simulink model "blockdemo"  (Simulink 6.3)
settings: Solver=ode45  StartTime=0.0  StopTime=30  RelTol=1e-3
InitFcn:
  | %% DSPBuilder Start
  | alt_dspbuilder_update_model(bdroot)
  | %% DSPBuilder End
libraries: allblocks_alteradspbuilder2 x7
settings Model: Creator=cpurcell  LastModifiedBy=delphick
settings DebuggingCC: MultiTaskDSMMsg=error

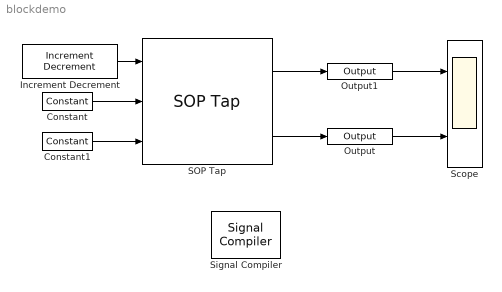
== system blockdemo ==
  Constant : allblocks_alteradspbuilder2/Constant  mask_cst=3.25  BusType=Signed Fractional  bwl=4  bwr=4  SpecifyClock=off
  Constant1 : allblocks_alteradspbuilder2/Constant  mask_cst=-1.75  BusType=Signed Fractional  bwl=4  bwr=4  SpecifyClock=off
  Increment Decrement : allblocks_alteradspbuilder2/Increment Decrement  BusType=Signed Fractional  bwl=2  bwr=2  SpecifyClock=off  clr_value=0  direction=Increment  phase_selection=1  use_ena=off  use_sclr=off
  Output : allblocks_alteradspbuilder2/Output  iofile=C:\workspace_clean\Documentation\DesignExamples\Tutorials\UnitBlocks\Arithmetic\SOPTap\tb_blockdemo\blockdemo_Output.capture  BusType=Inferred  bwl=8  bwr=0  PORTTYPE=Output
  Output1 : allblocks_alteradspbuilder2/Output  iofile=C:\workspace_clean\Documentation\DesignExamples\Tutorials\UnitBlocks\Arithmetic\SOPTap\tb_blockdemo\blockdemo_Output1.capture  BusType=Inferred  bwl=8  bwr=0  PORTTYPE=Output
  SOP Tap : allblocks_alteradspbuilder2/SOP Tap  BusType=Signed Fractional  bwl=4  bwr=4  number_of_taps=2  use_ena=off  use_aclr=off
  Scope : Scope  NumInputPorts=2
      settings: TimeRange=30  YMin=-10~-2  YMax=4~2
  Signal Compiler : allblocks_alteradspbuilder2/Signal Compiler  DeviceFamily=Stratix IV  DeviceName=AUTO  EnableSignalTap=off  SignalTapDepth=128  UseBoardBlock=off  StpUseDefaultClock=on  StpClock=clock
  wires:
  Increment Decrement/1 -> SOP Tap/1
  Constant/1 -> SOP Tap/2
  Constant1/1 -> SOP Tap/3
  SOP Tap/1 -> Output1/1
  SOP Tap/2 -> Output/1
  Output1/1 -> Scope/1
  Output/1 -> Scope/2
